simulink model "Q2"  (R2020b)
settings: Solver=VariableStepAuto  StartTime=0.0  StopTime=60  RelTol=1e-3
InitFcn:
  | H = 5;
  | Sb = 10000;
  | f0 = 50;
  | W0 = 100
  | DL = 1/200;
  | dPLoad = +1000
undefined symbols (not defined in the file): R, Tturb
Description:
  | Model of power system witthout control
  | Cretaed by Professor Francisco Gonzalez-Longatt
  | March 2021
settings Model: ModifiedHistory=Version 1: Created by Professor F. Gonzalez-Longatt 9 March 2021  Creator=fglon  LastModifiedBy=Dhanush Wagle

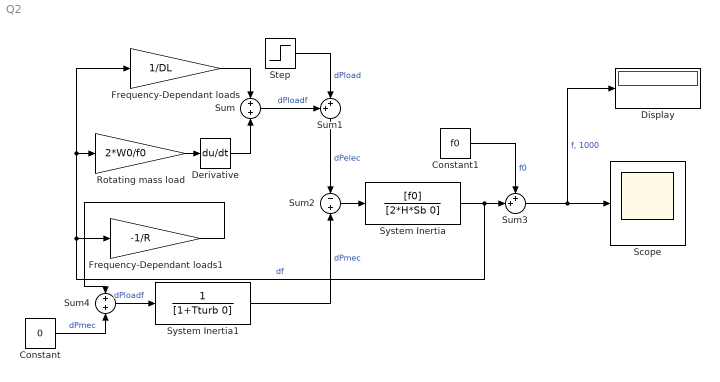
== system Q2 ==
  Constant : Constant  Value=0
  Constant1 : Constant  Value=f0
  Derivative : Derivative
  Display : Display
  Frequency-Dependant loads : Gain  Gain=1/DL
  Frequency-Dependant loads1 : Gain  Gain=-1/R
  Rotating mass load : Gain  Gain=2*W0/f0
  Scope : Scope
  Step : Step  After=100  SampleTime=0
  Sum : Sum  Inputs=+|+
  Sum1 : Sum  Inputs=++|
  Sum2 : Sum  Inputs=-|+
  Sum3 : Sum  Inputs=++|
  Sum4 : Sum  Inputs=+|+
  System Inertia : TransferFcn  Numerator=[f0]  Denominator=[2*H*Sb 0]
  System Inertia1 : TransferFcn  Denominator=[1+Tturb 0]
  wires:
  Rotating mass load/1 -> Derivative/1
  Derivative/1 -> Sum/2
  Frequency-Dependant loads/1 -> Sum/1
  Sum/1 -> Sum1/1  "dPloadf"
  Step/1 -> Sum1/2  "dPload"
  Sum1/1 -> Sum2/1  "dPelec"
  Sum2/1 -> System Inertia/1
  System Inertia/1 -> Frequency-Dependant loads1/1, Frequency-Dependant loads/1, Rotating mass load/1, Sum3/2  "df"
  Constant1/1 -> Sum3/1  "f0"
  Sum4/1 -> System Inertia1/1  "dPloadf"
  Constant/1 -> Sum4/2  "dPmec"
  System Inertia1/1 -> Sum2/2  "dPmec"
  Frequency-Dependant loads1/1 -> Sum4/1
  Sum3/1 -> Display/1, Scope/1  "f, 1000"
